simulink model "Generator_Motor_Test_System"  (R2019b)
settings: Solver=FixedStepAuto  StartTime=0.0  StopTime=10.0  FixedStep=.01  RelTol=1e-3
libraries: Lib_PFSys_GenericGenerator_TMATS x1, Lib_PFSys_GenericMotor_TMATS x1, Lib_PFSys_Inverter_TMATS x1, Lib_Solve_SSNRSolverJC_TMATS x1
settings Model: Creator=mebell  LastModifiedBy=mebell

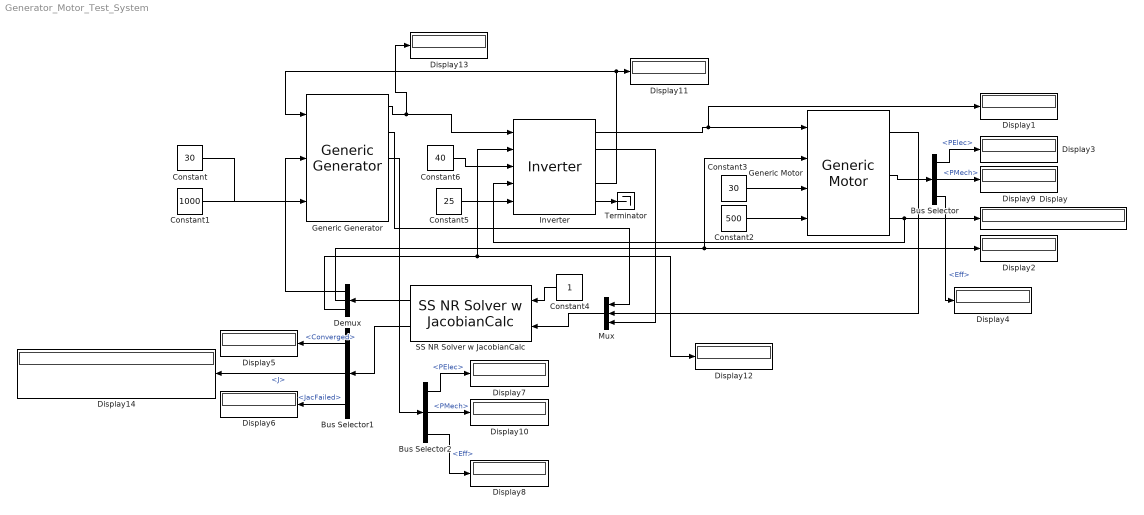
== system Generator_Motor_Test_System ==
  Bus Selector : BusSelector  OutputSignals=PElec,PMech,Eff
  Bus Selector1 : BusSelector  OutputSignals=Converged,J,JacFailed
  Bus Selector2 : BusSelector  OutputSignals=PElec,PMech,Eff
  Constant : Constant  Value=30
  Constant1 : Constant  Value=1000
  Constant2 : Constant  Value=500
  Constant3 : Constant  Value=30
  Constant4 : Constant
  Constant5 : Constant  Value=25
  Constant6 : Constant  Value=40
  Demux : Demux  Outputs=3
  Display{,1..14} (15 alike) : Display
      Display settings: Format=short_e
  Generic Generator : Lib_PFSys_GenericGenerator_TMATS/Generic Generator  X_C_SpeedVec_M=[0.0 0.1 1.0]  Y_C_TorqueVec_M=[0.0 0.1 1.0]  T_C_EffArray_M=[0.5 0.5 0.5; 0.5 1.0 1.0; 0.5 1.0 1.0]  Z_M=0.01  Ke_M=0.5
  Generic Motor : Lib_PFSys_GenericMotor_TMATS/Generic Motor  X_C_SpeedVec_M=[0.0 0.1 1.0]  Y_C_TorqueVec_M=[0.0 0.1 1.0]  T_C_EffArray_M=[0.5 0.5 0.5; 0.5 1.0 1.0; 0.5 1.0 1.0]  Z_M=0.01
  "Inverter " : Lib_PFSys_Inverter_TMATS/Inverter    Hz_to_V_M=22  X_C_VoltageVec_M=[0.0 0.1 1.0]  Y_C_CurrentVec_M=[0.0 0.1 1.0]  T_C_EffArray_M=[0.5 0.5 0.5; 0.5 1.0 1.0; 0.5 1.0 1.0]  Pdis_M=1
  Mux : Mux  Inputs=3
  SS NR Solver w JacobianCalc : Lib_Solve_SSNRSolverJC_TMATS/SS NR Solver w JacobianCalc  SJac_Per_M=[0.01 0.01 0.01;-0.01 -0.01 -0.01]  SNR_IC_M=[2; 3; 4]  SNR_DX_M=5  SNR_Mx_M=100000  SNR_Mn_M=0.00001  SJacobianAttempts_M=50  Cond_Limits_M=0.01
  Terminator : Terminator
  wires:
  Generic Generator/2 -> Mux/1
  Generic Motor/1 -> Mux/2
  Mux/1 -> SS NR Solver w JacobianCalc/2
  SS NR Solver w JacobianCalc/1 -> Demux/1
  Generic Motor/3 -> "Inverter "/4, Display/1
  Demux/2 -> Display2/1, Generic Motor/2
  Demux/1 -> Generic Generator/2
  Constant/1 -> Generic Generator/3
  Constant1/1 -> ?
  Constant2/1 -> Generic Motor/4
  Constant3/1 -> Generic Motor/3
  Constant4/1 -> SS NR Solver w JacobianCalc/1
  Generic Motor/2 -> Bus Selector/1
  Bus Selector/1 -> Display3/1  "<PElec>"
  Bus Selector/3 -> Display4/1  "<Eff>"
  SS NR Solver w JacobianCalc/2 -> Bus Selector1/1
  Bus Selector1/3 -> Display6/1  "<JacFailed>"
  Bus Selector1/1 -> Display5/1  "<Converged>"
  Bus Selector2/1 -> Display7/1  "<PElec>"
  Bus Selector2/3 -> Display8/1  "<Eff>"
  Generic Generator/3 -> Bus Selector2/1
  Bus Selector/2 -> Display9/1  "<PMech>"
  Bus Selector2/2 -> Display10/1  "<PMech>"
  "Inverter "/1 -> Display1/1, Generic Motor/1
  Generic Generator/1 -> Display13/1, "Inverter "/1
  "Inverter "/4 -> Generic Generator/1, Display11/1
  Constant5/1 -> "Inverter "/5
  "Inverter "/5 -> Terminator/1
  "Inverter "/2 -> Mux/3
  Demux/3 -> Display12/1, "Inverter "/2
  Constant6/1 -> "Inverter "/3
  Bus Selector1/2 -> Display14/1  "<J>"
